simulink model "dbl_xspec_xfer"  (R2021b)
settings: Solver=VariableStepAuto  StartTime=0.0  StopTime=2000  RelTol=1e-6
PreLoadFcn:
  | preload_fcn
StartFcn:
  | tic
StopFcn:
  | trun = toc
values from neighbouring files (symbols this model uses):
  BW = 10    [preload_fcn.m]
  Fs = OSR*BW    (= 25.6)    [preload_fcn.m]
  mag = squeeze(mag)    [preload_fcn.m]
  NFFT = 1024    [preload_fcn.m]
  phz = squeeze(phz)    [preload_fcn.m]
undefined symbols (not defined in the file or in its folder): dspblkcrossspectrumtfe
libraries: dsparch4 x4, dspsrcs4 x3, simulink_extras x1, dspspect3 x1, dspmathops x1
settings Model: SimulationMode=accelerator  NumberOfSteps=32000  Creator=kschutz  LastModifiedBy=kschutz

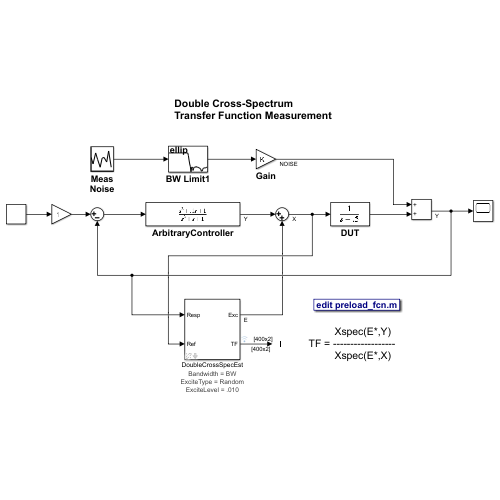
[thumbnail: Simulink's stored preview of the top-level diagram]
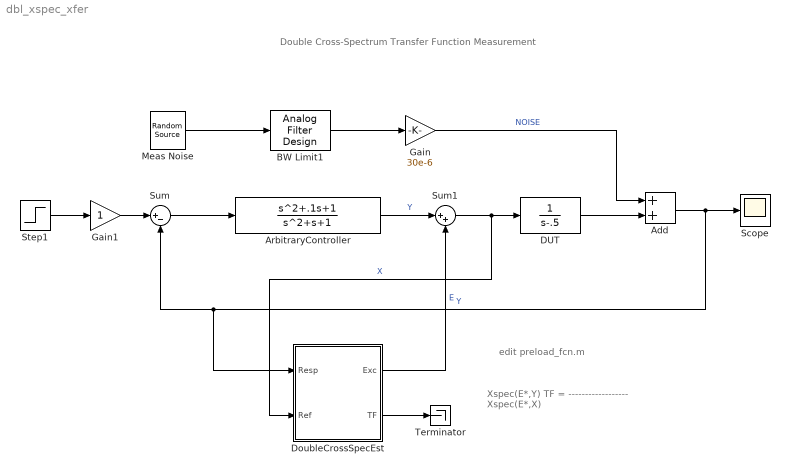
== system dbl_xspec_xfer ==
  note: Double Cross-Spectrum
      | Transfer Function Measurement
  note: edit preload_fcn.m
  note: Xspec(E*,Y)
      | TF = ------------------
      |          Xspec(E*,X)
  Add : Sum
  ArbitraryController : TransferFcn  Numerator=[1 .1 1]  Denominator=[1 1 1]
  BW Limit1 : dsparch4/Analog Filter Design  method=Elliptic  filttype=Lowpass  N=8  Wlo=2*pi*BW*10  Whi=80  Rp=2  Rs=80
  DUT : TransferFcn  Denominator=[1 -.5]
  DoubleCrossSpecEst : Subsystem  AncestorBlock=Kblocks/Analog Transfer Function Estimator  mask(Baseband Analog Transfer Function Estimator){BW=BW, Level=.010, ExcitationType=Random, Nfft=NFFT, Navg=100, HoldOff=100}
      mask prompts: BW "Bandwidth"; Level "Excitation Level"; ExcitationType "Excitation Type"; Nfft "FFT size"; Navg "Number of Averages"; HoldOff "Hold Off (seconds)"
      mask init:
      | % Select subset of FFT bins that are not aliased
      | % for output and display purposes.
      | % Said subset is based on the oversampling factor.
      | % Here we use a 2.56x oversampling factor.
      | % For example, for a 1024 point FFT size, the relatively
      | % alias free FFT bins would be bins 1 to 401.
      | % floor(1024/2.56) + 1 = 401.
      | OSR = 2.56;
      | AliasFree = floor(Nfft/OSR);
      | %debug_init_cmd
      | sel=get_param(gcb,'ExcitationType');
      | switch sel
      |     case 'Chirp'
      |         set_param([gcb,'/Excitation_Variant'],'LabelModeActiveChoice','excitation_type==1');
      |         set_param([gcb,'/TFE/DBL_XSPEC_EST/XSPEC_EST1'],'Window','Rectangular');
      |         set_param([gcb,'/TFE/DBL_XSPEC_EST/XSPEC_EST2'],'Window','Rectangular');
      |     case 'Random'
      |         set_param([gcb,'/Excitation_Variant'],'LabelModeActiveChoice','excitation_type==2');
      |         set_param([gcb,'/TFE/DBL_XSPEC_EST/XSPEC_EST1'],'Window','Hann');
      |         set_param([gcb,'/TFE/DBL_XSPEC_EST/XSPEC_EST2'],'Window','Hann');
      |     otherwise
      |         error(['Unknown excitation type in initialization command of Double Cross-Spectrum Estimator block = ',sel]);
      | end
      settings: AttributesFormatString=|
      | Bandwidth = %<BW>
      | ExciteType = %<ExcitationType>
      | ExciteLevel = %<Level>
      mask TypeOptions ExcitationType: Chirp | Random
  Gain : Gain  Gain=30e-6
  Gain1 : Gain
  Meas Noise : dspsrcs4/Random Source  SrcType=Gaussian  NormMethod=Ziggurat  CltLength=12  MinVal=0  MaxVal=.01  MeanVal=0  VarVal=1  RepMode=Specify seed  rawSeed=456  IsInherit=off  SampMode=Discrete  SampTime=1/Fs  SampFrame=1  DataType=Double  OutComplex=Real  OutputFrames=off
  Scope : Scope
  Step1 : Step  After=.005  SampleTime=0
  Sum : Sum  Inputs=|+-
  Sum1 : Sum  Inputs=|++
  Terminator : Terminator
  wires:
  Gain1/1 -> Sum/1
  DoubleCrossSpecEst/2(TF) -> Terminator/1
  Sum/1 -> ArbitraryController/1
  Step1/1 -> Gain1/1
  BW Limit1/1 -> Gain/1
  Gain/1 -> Add/1  "NOISE"
  DUT/1 -> Add/2
  Meas Noise/1 -> BW Limit1/1
  Sum1/1 -> DoubleCrossSpecEst/2(Ref), DUT/1  "X"
  ArbitraryController/1 -> Sum1/1  "Y"
  Add/1 -> DoubleCrossSpecEst/1(Resp), Sum/2, Scope/1  "Y"
  DoubleCrossSpecEst/1(Exc) -> Sum1/2  "E"

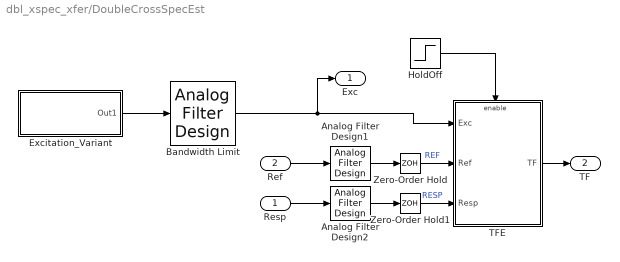
== system dbl_xspec_xfer/DoubleCrossSpecEst ==
  Resp : Inport
  Ref : Inport  Port=2
  Analog Filter Design1 : dsparch4/Analog Filter Design  method=Elliptic  filttype=Lowpass  N=8  Wlo=2*pi*BW  Whi=80  Rp=2  Rs=100
  Analog Filter Design2 : dsparch4/Analog Filter Design  method=Elliptic  filttype=Lowpass  N=8  Wlo=2*pi*BW  Whi=80  Rp=2  Rs=100
  Bandwidth Limit : dsparch4/Analog Filter Design  method=Elliptic  filttype=Lowpass  N=8  Wlo=2*pi*BW  Whi=80  Rp=2  Rs=100
  Excitation_Variant : Subsystem  Variant=on  VariantControlMode=label  LabelModeActiveChoice=excitation_type==2
  HoldOff : Step  Time=HoldOff  SampleTime=0
  TFE : Subsystem
  Zero-Order Hold : ZeroOrderHold  SampleTime=1/(OSR*BW)
  Zero-Order Hold1 : ZeroOrderHold  SampleTime=1/(OSR*BW)
  Exc : Outport
  TF : Outport  Port=2
  wires:
  Zero-Order Hold1/1 -> TFE/3(Resp)  "RESP"
  Analog Filter Design2/1 -> Zero-Order Hold1/1
  Resp/1 -> Analog Filter Design2/1
  Zero-Order Hold/1 -> TFE/2(Ref)  "REF"
  Ref/1 -> Analog Filter Design1/1
  Analog Filter Design1/1 -> Zero-Order Hold/1
  Excitation_Variant/1(Out1) -> Bandwidth Limit/1
  TFE/1(TF) -> TF/1
  HoldOff/1 -> TFE/Enable
  Bandwidth Limit/1 -> Exc/1, TFE/1(Exc)

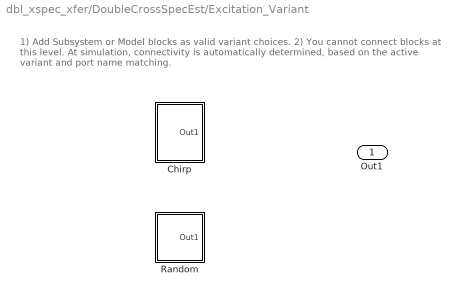
== system dbl_xspec_xfer/DoubleCrossSpecEst/Excitation_Variant ==
  note: 1) Add Subsystem or Model blocks as valid variant choices.
      | 2) You cannot connect blocks at this level. At simulation, connectivity is automatically
      | determined, based on the active variant and port name matching.
  Chirp : Subsystem  VariantControl=excitation_type==1
  Random : Subsystem  VariantControl=excitation_type==2
  Out1 : Outport

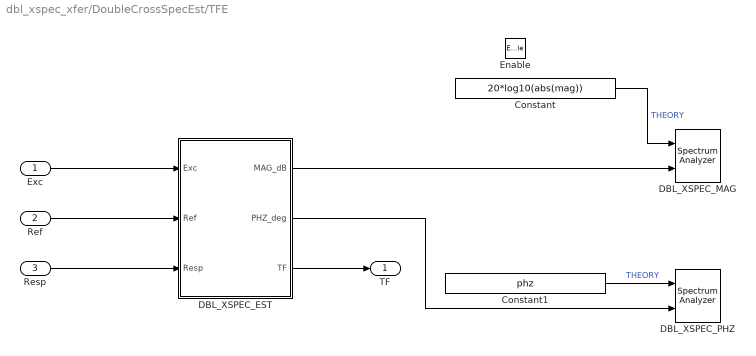
== system dbl_xspec_xfer/DoubleCrossSpecEst/TFE ==
  Exc : Inport
  Ref : Inport  Port=2
  Resp : Inport  Port=3
  Enable : EnablePort
  Constant : Constant  Value=20*log10(abs(mag))  VectorParams1D=off  SampleTime=(NFFT/OSR)/BW
  Constant1 : Constant  Value=phz  VectorParams1D=off  SampleTime=(NFFT/OSR)/BW
  DBL_XSPEC_EST : Subsystem
  DBL_XSPEC_MAG : SpectrumAnalyzer  NumInputPorts=2  IsFrequencyInputMode=1
  DBL_XSPEC_PHZ : SpectrumAnalyzer  NumInputPorts=2  IsFrequencyInputMode=1
  TF : Outport
  wires:
  DBL_XSPEC_EST/3(TF) -> TF/1
  DBL_XSPEC_EST/2(PHZ_deg) -> DBL_XSPEC_PHZ/2
  DBL_XSPEC_EST/1(MAG_dB) -> DBL_XSPEC_MAG/2
  Resp/1 -> DBL_XSPEC_EST/3(Resp)
  Ref/1 -> DBL_XSPEC_EST/2(Ref)
  Exc/1 -> DBL_XSPEC_EST/1(Exc)
  Constant/1 -> DBL_XSPEC_MAG/1  "THEORY"
  Constant1/1 -> DBL_XSPEC_PHZ/1  "THEORY"

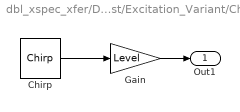
== system dbl_xspec_xfer/DoubleCrossSpecEst/Excitation_Variant/Chirp ==
  Chirp : dspsrcs4/Chirp  sweep=Linear  mode=Unidirectional  f0=0  f1=BW  t1=Nfft/(BW*2.56)  Tsweep=Nfft/(BW*2.56)  phase=3*pi/2  Ts=1/(2.56*BW)  spf=1  datatype=Double  OutputFrames=on
  Gain : Gain  Gain=Level
  Out1 : Outport
  wires:
  Gain/1 -> Out1/1
  Chirp/1 -> Gain/1

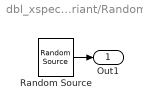
== system dbl_xspec_xfer/DoubleCrossSpecEst/Excitation_Variant/Random ==
  Random Source : dspsrcs4/Random Source  SrcType=Uniform  NormMethod=Ziggurat  CltLength=12  MinVal=-Level  MaxVal=Level  MeanVal=0  VarVal=1  RepMode=Specify seed  rawSeed=1  IsInherit=off  SampMode=Discrete  SampTime=1/(2.56*BW)  SampFrame=1  DataType=Double  OutComplex=Real  OutputFrames=off
  Out1 : Outport
  wires:
  Random Source/1 -> Out1/1

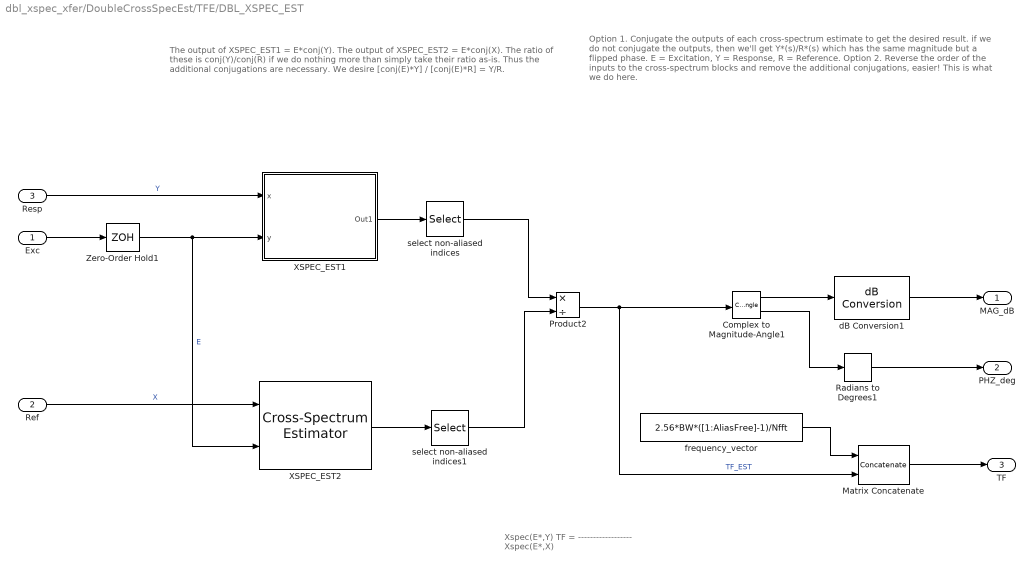
== system dbl_xspec_xfer/DoubleCrossSpecEst/TFE/DBL_XSPEC_EST ==
  note: Option 1. Conjugate the outputs of each cross-spectrum estimate to get the desired result. if we do not conjugate the outputs, then we'll get Y*(s)/R*(s) which has the same magnitude but a flipped phase. E = Excitation, Y = Response, R = Reference.
      |
      | Option 2. Reverse the order of the inputs to the cross-spectrum blocks and remove the additional conjugations, easier!
      | This is what we do here.
  note: The output of XSPEC_EST1 = E*conj(Y).
      | The output of XSPEC_EST2 = E*conj(X).
      | The ratio of these is conj(Y)/conj(R) if we do nothing more than
      | simply take their ratio as-is. Thus the additional conjugations
      | are necessary.
      | We desire [conj(E)*Y] / [conj(E)*R] = Y/R.
  note: Xspec(E*,Y)
      | TF = ------------------
      |          Xspec(E*,X)
  Exc : Inport
  Ref : Inport  Port=2
  Resp : Inport  Port=3
  Complex to Magnitude-Angle1 : ComplexToMagnitudeAngle
  Matrix Concatenate : Concatenate  Mode=Multidimensional array  ConcatenateDimension=2
  Product2 : Product  Inputs=*/  InputSameDT=on  SaturateOnIntegerOverflow=on  OutDataTypeStr=Inherit: Same as first input
  Radians to Degrees1 : simulink_extras/Transformations/Radians to Degrees
  XSPEC_EST1 : Subsystem  InitFcn=dspblkcrossspectrumtfe(gcb,'setup')  TreatAsAtomicUnit=on  mask(Cross-Spectrum Estimator){WindowMode=Specify on dialog, WindowLength=Nfft, Overlap=0, AveragingMethod=Running, ForgettingFactorPort=off, ForgettingFactor=0.9, SpectralAverages=Navg, FFTLengthSource=Property, FFTLength=Nfft, Window=Hann, SidelobeAttenuation=60, FrequencyRange=One-sided, InheritSampleRate=on, SampleRate=44100, SimulateUsing=Interpreted execution}
      mask prompts: WindowMode "dsp:SpectrumEstimation_BlockDialog:WindowMode_MP"; WindowLength "dsp:SpectrumEstimation_BlockDialog:WindowLength_MP"; Overlap "dsp:SpectrumEstimation_BlockDialog:Overlap_MP"; AveragingMethod "dsp:SpectrumEstimation_BlockDialog:AveragingMethod_MP"; ForgettingFactorPort "Specify forgetting factor from input port"; ForgettingFactor "Forgetting factor:"; SpectralAverages "dsp:SpectrumEstimation_BlockDialog:SpectralAverages_MP"; FFTLengthSource "dsp:SpectrumEstimation_BlockDialog:FFTLengthSource_MP"; FFTLength "dsp:SpectrumEstimation_BlockDialog:FFTLength_MP"; Window "dsp:SpectrumEstimation_BlockDialog:Window_MP"; SidelobeAttenuation "dsp:SpectrumEstimation_BlockDialog:SidelobeAttenuation_MP"; FrequencyRange "dsp:SpectrumEstimation_BlockDialog:FrequencyRange_MP"; InheritSampleRate "dsp:SpectrumEstimation_BlockDialog:InheritSampleRate_MP"; SampleRate "dsp:SpectrumEstimation_BlockDialog:SampleRate_MP"; SimulateUsing "dsp:SpectrumEstimation_BlockDialog:SimulateUsing_MP"
      mask help: dsp:SpectrumEstimation_BlockDialog:CrossSpectrumEstimator_MaskDesc
      mask init:
      | dspblkcrossspectrumtfe(gcb,'init');
      settings: AttributesFormatString=Window = %<Window>
      mask Help: eval('blocksethelp');
      mask TypeOptions WindowMode: dsp:SpectrumEstimation_BlockDialog:WindowLengthSourceEnum_SameAsInput | dsp:SpectrumEstimation_BlockDialog:WindowLengthSourceEnum_Dialog
      mask Callback WindowMode: dspblkcrossspectrumtfe(gcb,'dynamic','WindowMode')
      mask TypeOptions AveragingMethod: dsp:SpectrumEstimation_BlockDialog:AveragingMethodEnum_Running | dsp:SpectrumEstimation_BlockDialog:AveragingMethodEnum_Exponential
      mask Callback AveragingMethod: dspblkcrossspectrumtfe(gcb,'dynamic','AveragingMethod')
      mask TypeOptions ForgettingFactorPort: Cross-Spectrum Estimator/ForgettingFactorPort
      mask Callback ForgettingFactorPort: dspblkcrossspectrumtfe(gcb,'dynamic','ForgettingFactorPort')
      mask TypeOptions ForgettingFactor: Cross-Spectrum Estimator/ForgettingFactor
      mask TypeOptions FFTLengthSource: dsp:SpectrumEstimation_BlockDialog:Auto | dsp:SpectrumEstimation_BlockDialog:Property
      mask Callback FFTLengthSource: dspblkcrossspectrumtfe(gcb,'dynamic','FFTLengthSource')
      mask TypeOptions Window: dsp:SpectrumEstimation_BlockDialog:WindowEnum_Chebyshev | dsp:SpectrumEstimation_BlockDialog:WindowEnum_FlatTop | dsp:SpectrumEstimation_BlockDialog:WindowEnum_Hamming | dsp:SpectrumEstimation_BlockDialog:WindowEnum_Hann | dsp:SpectrumEstimation_BlockDialog:WindowEnum_Kaiser | dsp:SpectrumEstimation_BlockDialog:WindowEnum_Rectangular
      mask Callback Window: dspblkcrossspectrumtfe(gcb,'dynamic','Window')
      mask TypeOptions FrequencyRange: dsp:SpectrumEstimation_BlockDialog:FrequencyRangeEnum_OneSided | dsp:SpectrumEstimation_BlockDialog:FrequencyRangeEnum_TwoSided | dsp:SpectrumEstimation_BlockDialog:FrequencyRangeEnum_Centered
      mask Callback InheritSampleRate: dspblkcrossspectrumtfe(gcb,'dynamic','InheritSampleRate')
      mask TypeOptions SimulateUsing: dsp:SpectrumEstimation_BlockDialog:SimulateUsingEnum_CG | dsp:SpectrumEstimation_BlockDialog:SimulateUsingEnum_Interpreted
      mask DialogControl WindowMode Prompt: Window length source:
      mask DialogControl WindowLength Prompt: Window length:
      mask DialogControl Overlap Prompt: Window overlap (%):
      mask DialogControl AveragingMethod Prompt: Averaging method:
      mask DialogControl SpectralAverages Prompt: Number of spectral averages:
      mask DialogControl FFTLengthSource Prompt: FFT length source:
      mask DialogControl FFTLength Prompt: FFT length:
      mask DialogControl Window Prompt: Window function:
      mask DialogControl SidelobeAttenuation Prompt: Sidelobe attenuation of window (dB):
      mask DialogControl FrequencyRange Prompt: Frequency range:
      mask DialogControl InheritSampleRate Prompt: Inherit sample rate from input
      mask DialogControl SampleRate Prompt: Sample rate (Hz):
      mask DialogControl SimulateUsing Prompt: Simulate using
      mask Display:
      | fprintf(getString(message('dsp:system:SpectrumEstimatorBase:CrossSpectrumEstimatorIcon')))
      | blk = gcbh;
      | port_label('input', 1, 'x')
      | port_label('input', 2, 'y')
      | if strcmp(get_param(blk,'ForgettingFactorPort'),'on')
      |   port_label('input', 3, 'lambda');
      | end
  XSPEC_EST2 : dspspect3/Cross-Spectrum Estimator  WindowMode=Specify on dialog  WindowLength=Nfft  Overlap=0  AveragingMethod=Running  ForgettingFactorPort=off  ForgettingFactor=0.9  SpectralAverages=Navg  FFTLengthSource=Property  FFTLength=Nfft  Window=Hann  SidelobeAttenuation=60  FrequencyRange=One-sided  InheritSampleRate=on  SampleRate=44100  SimulateUsing=Interpreted execution
      settings: AttributesFormatString=Window = %<Window>  SourceProductBaseCode=DS
  Zero-Order Hold1 : ZeroOrderHold  SampleTime=1/(OSR*BW)
  dB Conversion1 : dspmathops/dB Conversion  dBtype=dB  intype=Amplitude  R=1  fuzz=off
  frequency_vector : Constant  Value=2.56*BW*([1:AliasFree]-1)/Nfft
  select non-aliased indices : Selector  NumberOfDimensions=2  InputPortWidth=3  IndexOptions=Index vector (dialog),Select all  Indices=[1:AliasFree ],1  OutputSizes=1,1
  select non-aliased indices1 : Selector  NumberOfDimensions=2  InputPortWidth=3  IndexOptions=Index vector (dialog),Select all  Indices=[1:AliasFree ],1  OutputSizes=1,1
  MAG_dB : Outport
  PHZ_deg : Outport  Port=2
  TF : Outport  Port=3
  wires:
  Ref/1 -> XSPEC_EST2/1  "X"
  Resp/1 -> XSPEC_EST1/1(x)  "Y"
  select non-aliased indices/1 -> Product2/1
  select non-aliased indices1/1 -> Product2/2
  frequency_vector/1 -> Matrix Concatenate/1
  Matrix Concatenate/1 -> TF/1
  Radians to Degrees1/1 -> PHZ_deg/1
  Zero-Order Hold1/1 -> XSPEC_EST1/2(y), XSPEC_EST2/2  "E"
  Product2/1 -> Matrix Concatenate/2, Complex to Magnitude-Angle1/1  "TF_EST"
  Complex to Magnitude-Angle1/1 -> dB Conversion1/1
  dB Conversion1/1 -> MAG_dB/1
  Complex to Magnitude-Angle1/2 -> Radians to Degrees1/1
  XSPEC_EST2/1 -> select non-aliased indices1/1
  XSPEC_EST1/1(Out1) -> select non-aliased indices/1
  Exc/1 -> Zero-Order Hold1/1

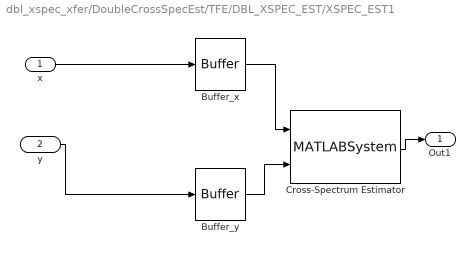
== system dbl_xspec_xfer/DoubleCrossSpecEst/TFE/DBL_XSPEC_EST/XSPEC_EST1 ==
  x : Inport
  y : Inport  Port=2
  Buffer_x : Buffer  N=WindowLength  OutputFrames=off
  Buffer_y : Buffer  N=WindowLength  OutputFrames=off
  Cross-Spectrum Estimator : MATLABSystem  System=dsp.simulink.CrossSpectrumEstimator  AveragingMethod=Running  SpectralAverages=100  ForgettingFactorPort=off  ForgettingFactor=ForgettingFactor  FFTLengthSource=Property  FFTLength=1024  Window=Hann  SidelobeAttenuation=60  FrequencyRange=onesided  InheritSampleRate=on  SampleRate=1  SimulateUsing=Interpreted execution
      mask Type: dsp.simulink.CrossSpectrumEstimator
      mask Display:
      | disp(['Cross-Spectrum' char(10) 'Estimator']);
      | port_label('input',1,'x');
      | port_label('input',2,'y');
  Out1 : Outport  VectorParamsAs1DForOutWhenUnconnected=off
  wires:
  Cross-Spectrum Estimator/1 -> Out1/1
  y/1 -> Buffer_y/1
  Buffer_y/1 -> Cross-Spectrum Estimator/2
  Buffer_x/1 -> Cross-Spectrum Estimator/1
  x/1 -> Buffer_x/1
